simulink subsystem "PID_anti_windup"  (R2024a)
settings: Solver=VariableStepAuto  StartTime=0.0  StopTime=10.0  RelTol=1e-3
undefined symbols (not defined in the file or in its folder): K, u_eq
settings Model: Creator=Bocchio  LastModifiedBy=Bocchio

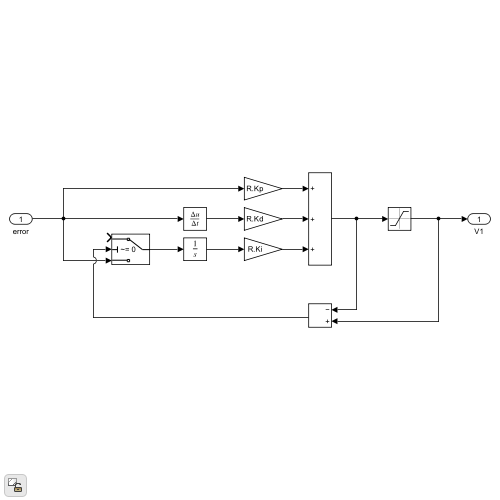
[thumbnail: Simulink's stored preview of the top-level diagram]
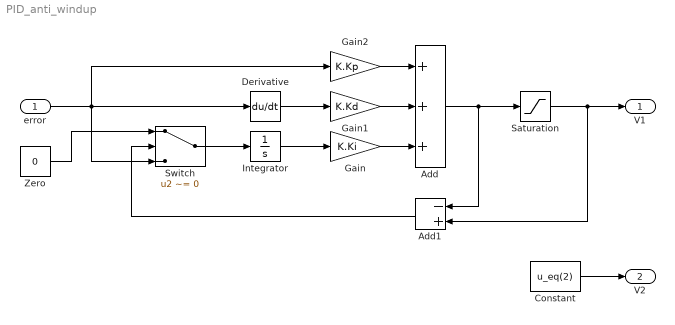
== system PID_anti_windup ==
  error : Inport
  Add : Sum  Inputs=+++
  Add1 : Sum  Inputs=-+
  Constant : Constant  Value=u_eq(2)
  Derivative : Derivative
  Gain : Gain  Gain=K.Ki
  Gain1 : Gain  Gain=K.Kd
  Gain2 : Gain  Gain=K.Kp
  Integrator : Integrator
  Saturation : Saturate  UpperLimit=1  LowerLimit=0
  Switch : Switch  Criteria=u2 ~= 0  SaturateOnIntegerOverflow=off  InputSameDT=off
  Zero : Constant  Value=0  OutDataTypeStr=Inherit: Inherit via back propagation
  V1 : Outport
  V2 : Outport  Port=2
  wires:
  Add1/1 -> Switch/2
  Saturation/1 -> Add1/2, V1/1
  error/1 -> Derivative/1, Switch/3, Gain2/1
  Add/1 -> Add1/1, Saturation/1
  Switch/1 -> Integrator/1
  Gain2/1 -> Add/1
  Gain1/1 -> Add/2
  Gain/1 -> Add/3
  Derivative/1 -> Gain1/1
  Integrator/1 -> Gain/1
  Constant/1 -> V2/1
  Zero/1 -> Switch/1
